simulink model "SISTEMA_DI_CONTROLLO"  (R2018a)
settings: Solver=VariableStepAuto  StartTime=0.0  StopTime=10.0  RelTol=1e-3
undefined symbols (not defined in the file or in its folder): Pose, Twist
libraries: robotlib x5
settings Model: Creator=root  LastModifiedBy=root

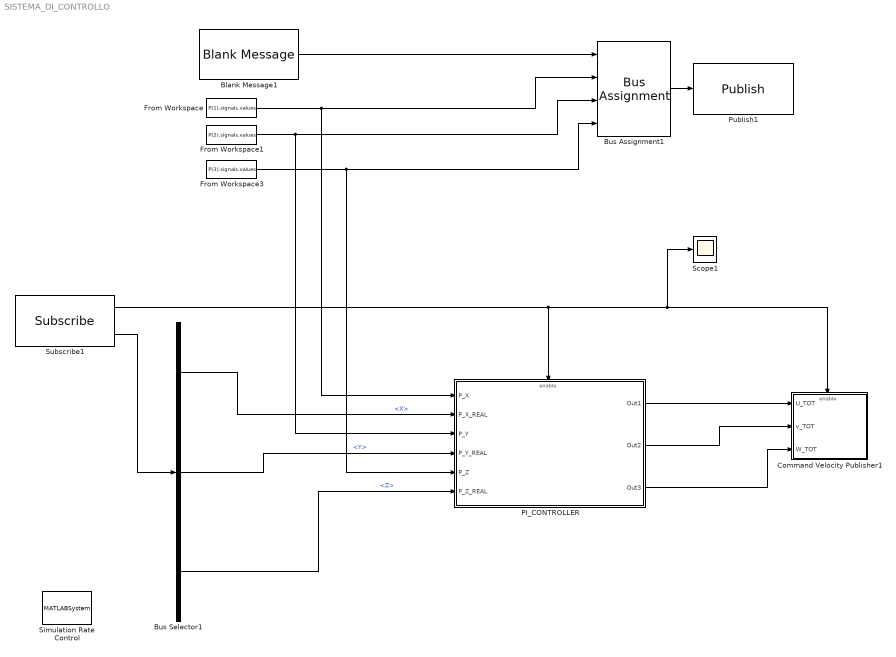
== system SISTEMA_DI_CONTROLLO ==
  " PI_CONTROLLER " : Subsystem  TreatAsAtomicUnit=on
  Blank Message1 : robotlib/Blank Message  SourceLibraryInfo=This block requires Robotics System Toolbox  messageType=geometry_msgs/PoseStamped  SampleTime=inf
      settings: SourceProductBaseCode=RO
  Bus Assignment1 : BusAssignment  AssignedSignals=Pose.Position.X,Pose.Position.Y,Pose.Position.Z
  Bus Selector1 : BusSelector  OutputSignals=Pose.Position.X,Pose.Position.Y,Pose.Position.Z
  Command Velocity Publisher1 : Subsystem
  From Workspace : FromWorkspace  VariableName=P(1).signals.values  SampleTime=0
  From Workspace1 : FromWorkspace  VariableName=P(2).signals.values  SampleTime=0
  From Workspace3 : FromWorkspace  VariableName=P(3).signals.values  SampleTime=0
  Publish1 : robotlib/Publish  SourceLibraryInfo=This block requires Robotics System Toolbox  topicSource=Select from ROS network  topic=/ual/set_pose  messageType=geometry_msgs/PoseStamped  messageQueueLength=1
      settings: SourceProductBaseCode=RO
  Scope1 : Scope
  Simulation Rate Control : MATLABSystem  System=ExampleHelperSimulationRateControl  SampleTime=0.02
      mask Type: ExampleHelperSimulationRateControl
      mask Display: disp('Rate Control');
  Subscribe1 : robotlib/Subscribe  SourceLibraryInfo=This block requires Robotics System Toolbox  topicSource=Select from ROS network  topic=/ual/pose  messageType=geometry_msgs/PoseStamped  sampleTime=inf  messageQueueLength=1
      settings: SourceProductBaseCode=RO
  wires:
  From Workspace/1 -> " PI_CONTROLLER "/1(P_X), Bus Assignment1/2
  Blank Message1/1 -> Bus Assignment1/1
  From Workspace1/1 -> " PI_CONTROLLER "/3(P_Y), Bus Assignment1/3
  Bus Assignment1/1 -> Publish1/1
  From Workspace3/1 -> " PI_CONTROLLER "/5(P_Z), Bus Assignment1/4
  Bus Selector1/2 -> " PI_CONTROLLER "/4(P_Y_REAL)  "<Y>"
  Bus Selector1/1 -> " PI_CONTROLLER "/2(P_X_REAL)  "<X>"
  Bus Selector1/3 -> " PI_CONTROLLER "/6(P_Z_REAL)  "<Z>"
  Subscribe1/2 -> Bus Selector1/1
  Subscribe1/1 -> Scope1/1, Command Velocity Publisher1/Enable, " PI_CONTROLLER "/Enable
  " PI_CONTROLLER "/1(Out1) -> Command Velocity Publisher1/1(U_TOT)
  " PI_CONTROLLER "/2(Out2) -> Command Velocity Publisher1/2(v_TOT)
  " PI_CONTROLLER "/3(Out3) -> Command Velocity Publisher1/3(W_TOT)

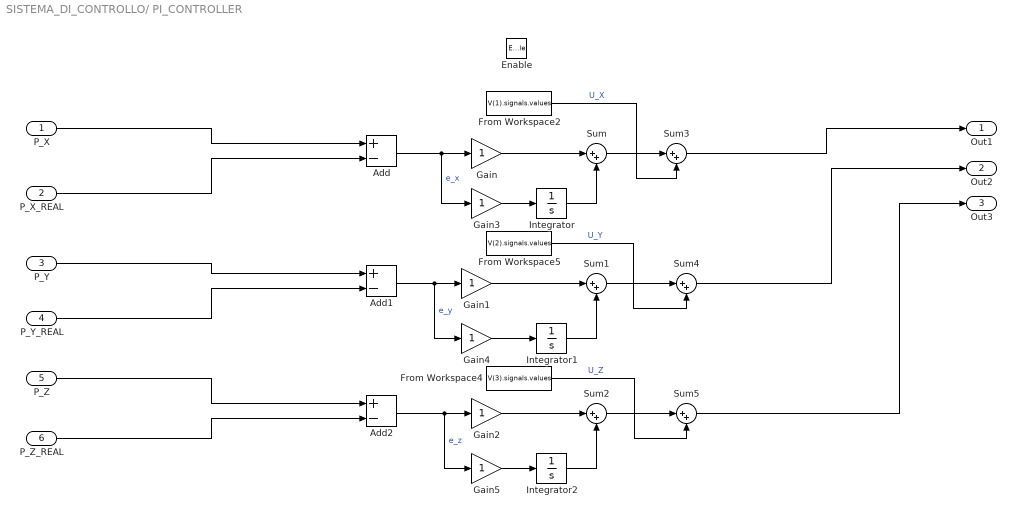
== system SISTEMA_DI_CONTROLLO/ PI_CONTROLLER  ==
  P_X : Inport
  P_X_REAL : Inport  Port=2
  P_Y : Inport  Port=3
  P_Y_REAL : Inport  Port=4
  P_Z : Inport  Port=5
  P_Z_REAL : Inport  Port=6
  Enable : EnablePort
  Add : Sum  Inputs=+-
  Add1 : Sum  Inputs=+-
  Add2 : Sum  Inputs=+-
  From Workspace2 : FromWorkspace  VariableName=V(1).signals.values  SampleTime=0
  From Workspace4 : FromWorkspace  VariableName=V(3).signals.values  SampleTime=0
  From Workspace5 : FromWorkspace  VariableName=V(2).signals.values  SampleTime=0
  Gain{,1..5} (6 alike) : Gain
  Integrator : Integrator
  Integrator1 : Integrator
  Integrator2 : Integrator
  Sum{,1..5} (6 alike) : Sum  Inputs=|++
  Out1 : Outport
  Out2 : Outport  Port=2
  Out3 : Outport  Port=3
  wires:
  Gain1/1 -> Sum1/1
  Sum2/1 -> Sum5/1
  Integrator1/1 -> Sum1/2
  Integrator/1 -> Sum/2
  Add/1 -> Gain3/1, Gain/1  "e_x"
  Integrator2/1 -> Sum2/2
  Add1/1 -> Gain4/1, Gain1/1  "e_y"
  From Workspace4/1 -> Sum5/2  "U_Z"
  Sum1/1 -> Sum4/1
  From Workspace2/1 -> Sum3/2  "U_X"
  Gain5/1 -> Integrator2/1
  Gain2/1 -> Sum2/1
  Add2/1 -> Gain5/1, Gain2/1  "e_z"
  Gain4/1 -> Integrator1/1
  Gain3/1 -> Integrator/1
  Sum/1 -> Sum3/1
  From Workspace5/1 -> Sum4/2  "U_Y"
  Gain/1 -> Sum/1
  P_X/1 -> Add/1
  P_X_REAL/1 -> Add/2
  P_Y/1 -> Add1/1
  P_Y_REAL/1 -> Add1/2
  P_Z/1 -> Add2/1
  P_Z_REAL/1 -> Add2/2
  Sum3/1 -> Out1/1
  Sum4/1 -> Out2/1
  Sum5/1 -> Out3/1

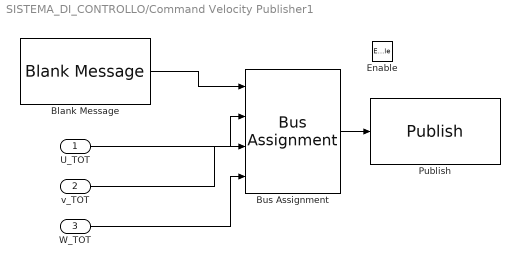
== system SISTEMA_DI_CONTROLLO/Command Velocity Publisher1 ==
  U_TOT : Inport
  v_TOT : Inport  Port=2
  W_TOT : Inport  Port=3
  Enable : EnablePort
  Blank Message : robotlib/Blank Message  SourceLibraryInfo=This block requires Robotics System Toolbox  messageType=geometry_msgs/TwistStamped  SampleTime=inf
      settings: SourceProductBaseCode=RO
  Bus Assignment : BusAssignment  AssignedSignals=Twist.Linear.X,Twist.Linear.Z,Twist.Linear.Y
  Publish : robotlib/Publish  SourceLibraryInfo=This block requires Robotics System Toolbox  topicSource=Select from ROS network  topic=/ual/set_velocity  messageType=geometry_msgs/TwistStamped  messageQueueLength=1
      settings: SourceProductBaseCode=RO
  wires:
  U_TOT/1 -> Bus Assignment/2
  v_TOT/1 -> Bus Assignment/3
  Bus Assignment/1 -> Publish/1
  Blank Message/1 -> Bus Assignment/1
  W_TOT/1 -> Bus Assignment/4
